simulink model "AplysiaFeedingSimulation - Copy"  (R2019b)
settings: Solver=FixedStepAuto  StartTime=0.0  StopTime=40  FixedStep=0.05  RelTol=1e-3
values from neighbouring files (symbols this model uses):
  A_hinge_Init = 0.05    [AplysiaFeedingNew.m]
  A_I2_Init = 0.05    [AplysiaFeedingNew.m]
  A_I3_anterior_Init = 0.05    [AplysiaFeedingNew.m]
  A_I3_Init = 0.05    [AplysiaFeedingNew.m]
  A_I4_Init = 0.05    [AplysiaFeedingNew.m]
  B20_Init = 0    [AplysiaFeedingNew.m]
  B31B32_Init = 1    [AplysiaFeedingNew.m]
  B38_Init = 1    [AplysiaFeedingNew.m]
  B40B30_Init = 0    [AplysiaFeedingNew.m]
  B4B5_Init = 0    [AplysiaFeedingNew.m]
  B64_Init = 0    [AplysiaFeedingNew.m]
  B6B9B3_Init = 0    [AplysiaFeedingNew.m]
  B7_Init = 0    [AplysiaFeedingNew.m]
  B8_Init = 0    [AplysiaFeedingNew.m]
  c_g = 1.0    (= 1)    [AplysiaFeedingNew.m]
  c_h = 1.0    (= 1)    [AplysiaFeedingNew.m]
  CBI2_Init = 1    [AplysiaFeedingNew.m]
  CBI3_Init = 0    [AplysiaFeedingNew.m]
  CBI4_Init = 0    [AplysiaFeedingNew.m]
  fixation_type_final = 10000    [AplysiaFeedingNew.m]
  fixation_type_initial = 10000    [AplysiaFeedingNew.m]
  K_sp_g = 0.1    [AplysiaFeedingNew.m]
  K_sp_h = 2.0    (= 2)    [AplysiaFeedingNew.m]
  max_hinge = 0.2    [AplysiaFeedingNew.m]
  max_I2 = 1.5    [AplysiaFeedingNew.m]
  max_I3 = 1    [AplysiaFeedingNew.m]
  max_I3ant = 0.6    [AplysiaFeedingNew.m]
  max_I4 = 1.75    [AplysiaFeedingNew.m]
  MCC_Init = 1    [AplysiaFeedingNew.m]
  mu_k_g = 0.3    [AplysiaFeedingNew.m]
  mu_k_h = 0.3    [AplysiaFeedingNew.m]
  mu_s_g = 0.4    [AplysiaFeedingNew.m]
  mu_s_h = 0.3    [AplysiaFeedingNew.m]
  P_I3_anterior_Init = 0    [AplysiaFeedingNew.m]
  P_I4_Init = 0    [AplysiaFeedingNew.m]
  postActivityExcitation_B40B30 = 3    [AplysiaFeedingNew.m]
  seaweed_strength = 10    [AplysiaFeedingNew.m]
  sens_chemical_lips_final = 10000    [AplysiaFeedingNew.m]
  sens_chemical_lips_initial = 10000    [AplysiaFeedingNew.m]
  sens_mechanical_grasper_final = 10000    [AplysiaFeedingNew.m]
  sens_mechanical_grasper_initial = 10000    [AplysiaFeedingNew.m]
  sens_mechanical_lips_final = 10000    [AplysiaFeedingNew.m]
  sens_mechanical_lips_initial = 10000    [AplysiaFeedingNew.m]
  sensory_trigger_time = 10000    [AplysiaFeedingNew.m]
  stim_B4B5_trigger_time_end = 10000    [AplysiaFeedingNew.m]
  stim_B4B5_trigger_time_start = 10000    [AplysiaFeedingNew.m]
  stim_CBI2_trigger_time_end = 10000    [AplysiaFeedingNew.m]
  stim_CBI2_trigger_time_start = 10000    [AplysiaFeedingNew.m]
  T_hinge_Init = 0    [AplysiaFeedingNew.m]
  T_I2_Init = 0.05    [AplysiaFeedingNew.m]
  T_I3_Init = 0.05    [AplysiaFeedingNew.m]
  tau_hinge = 1.0/sqrt(2)    [AplysiaFeedingNew.m]
  tau_I2_egestion = 1.4*1/sqrt(2)    [AplysiaFeedingNew.m]
  tau_I2_ingestion = 0.5*1/sqrt(2)    [AplysiaFeedingNew.m]
  tau_I3 = 1.0/sqrt(2)    [AplysiaFeedingNew.m]
  tau_I3anterior = 2.0/sqrt(2)    [AplysiaFeedingNew.m]
  tau_I4 = 1.0/sqrt(2)    [AplysiaFeedingNew.m]
  thresh_B31_bite_off = 0.55    [AplysiaFeedingNew.m]
  thresh_B31_bite_on = 0.9    [AplysiaFeedingNew.m]
  thresh_B31_reject_off = 0.6    [AplysiaFeedingNew.m]
  thresh_B31_reject_on = 0.89    [AplysiaFeedingNew.m]
  thresh_B31_swallow_off = 0.4    [AplysiaFeedingNew.m]
  thresh_B31_swallow_on = 0.75    [AplysiaFeedingNew.m]
  thresh_B4B5_protract = 0.7    [AplysiaFeedingNew.m]
  thresh_B64_bite_protract = 0.89    [AplysiaFeedingNew.m]
  thresh_B64_reject_protract = 0.5    [AplysiaFeedingNew.m]
  thresh_B64_swallow_protract = 0.4    [AplysiaFeedingNew.m]
  thresh_B6B9B3_bite_pressure = 0.2    [AplysiaFeedingNew.m]
  thresh_B6B9B3_reject_pressure = 0.75    [AplysiaFeedingNew.m]
  thresh_B6B9B3_swallow_pressure = 0.25    [AplysiaFeedingNew.m]
  unbroken_Init = 1    [AplysiaFeedingNew.m]
  use_hypothesized_connections = 0    [AplysiaFeedingNew.m]
  x_g_Init = 0.1    [AplysiaFeedingNew.m]
  x_gh_ref = 0.4    [AplysiaFeedingNew.m]
  x_h_Init = 0    [AplysiaFeedingNew.m]
  x_h_ref = 0.0    (= 0)    [AplysiaFeedingNew.m]
(part 2 of 2)

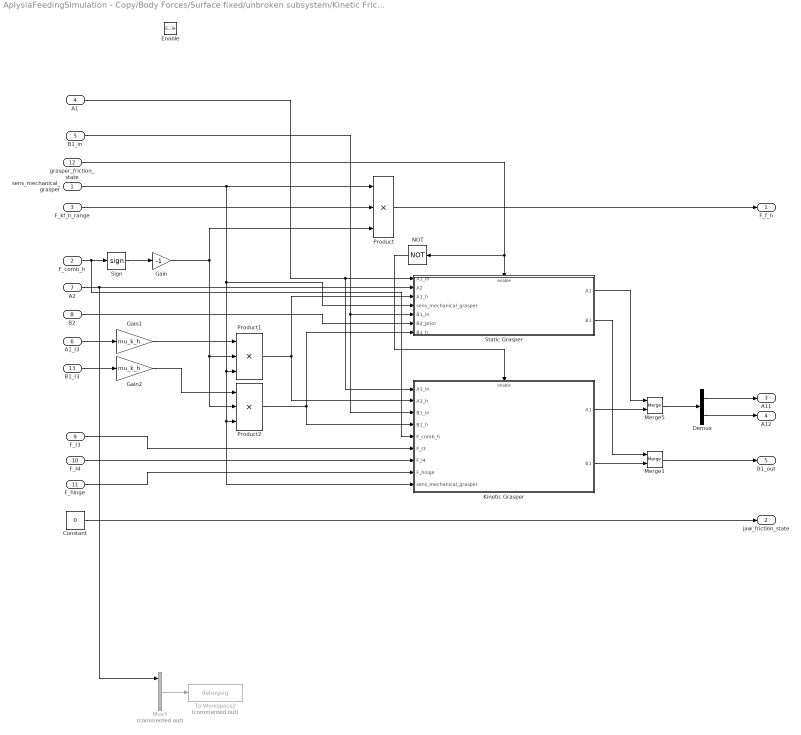
== system AplysiaFeedingSimulation - Copy/Body Forces/Surface fixed/unbroken subsystem/Kinetic Friction Behavior ==
  sens_mechanical_grasper : Inport
  F_comb_h : Inport  Port=2
  F_kf_h_range : Inport  Port=3
  A1 : Inport  Port=4
  B1_in : Inport  Port=5
  A1_I3 : Inport  Port=6
  A2 : Inport  Port=7
  B2 : Inport  Port=8
  F_I3 : Inport  Port=9
  F_I4 : Inport  Port=10
  F_hinge : Inport  Port=11
  grasper_friction_state : Inport  Port=12
  B1_I3 : Inport  Port=13
  Enable : EnablePort
  Constant : Constant  Value=0
  Demux : Demux  Outputs=2
  Gain : Gain  Gain=-1
  Gain1 : Gain  Gain=mu_k_h
  Gain2 : Gain  Gain=mu_k_h
  Kinetic Grasper : Subsystem
  Merge1 : Merge
  Merge5 : Merge
  Mux3 : Mux  Commented=on
  NOT : Logic  Operator=NOT  IconShape=distinctive  AllPortsSameDT=off  OutDataTypeStr=boolean
  Product : Product  Inputs=3
  Product1 : Product  Inputs=3
  Product2 : Product  Inputs=3
  Sign : Signum
  Static Grasper : Subsystem
  To Workspace2 : ToWorkspace  Commented=on  VariableName=debugsig  SaveFormat=Structure With Time  SampleTime=-1
  F_f_h : Outport
  jaw_friction_state : Outport  Port=2
  A11 : Outport  Port=3
  A12 : Outport  Port=4
  B1_out : Outport  Port=5
  wires:
  Constant/1 -> jaw_friction_state/1
  F_comb_h/1 -> Kinetic Grasper/5(F_comb_h), Sign/1
  Product/1 -> F_f_h/1
  F_kf_h_range/1 -> Product/2
  sens_mechanical_grasper/1 -> Static Grasper/4(sens_mechanical_grasper), Kinetic Grasper/9(sens_mechanical_grasper), Product2/3, Product1/3, Product/1
  Sign/1 -> Gain/1
  Gain/1 -> Product2/2, Product1/2, Product/3
  A1_I3/1 -> Gain1/1
  Gain1/1 -> Product1/1
  Merge5/1 -> Demux/1
  Demux/1 -> A11/1
  Demux/2 -> A12/1
  Static Grasper/1(A1) -> Merge5/1
  Kinetic Grasper/1(A1) -> Merge5/2
  Merge1/1 -> B1_out/1
  Kinetic Grasper/2(B1) -> Merge1/2
  Static Grasper/2(B1) -> Merge1/1
  A1/1 -> Kinetic Grasper/1(A1_in), Static Grasper/1(A1_in)
  B1_in/1 -> Static Grasper/5(B1_in), Kinetic Grasper/3(B1_in)
  B2/1 -> Static Grasper/6(B2_prior)
  F_hinge/1 -> Kinetic Grasper/8(F_hinge)
  F_I4/1 -> Kinetic Grasper/7(F_I4)
  F_I3/1 -> Kinetic Grasper/6(F_I3)
  grasper_friction_state/1 -> NOT/1, Static Grasper/Enable
  NOT/1 -> Kinetic Grasper/Enable
  Product1/1 -> Kinetic Grasper/2(A1_h), Static Grasper/3(A1_h)
  B1_I3/1 -> Gain2/1
  Gain2/1 -> Product2/1
  Product2/1 -> Kinetic Grasper/4(B1_h), Static Grasper/7(B1_h)
  Mux3/1 -> To Workspace2/1
  A2/1 -> Mux3/1, Static Grasper/2(A2)

== system AplysiaFeedingSimulation - Copy/Body Forces/Surface fixed/unbroken subsystem/Static Friction Behavior ==
  sens_mechanical_grasper : Inport
  F_comb_h : Inport  Port=2
  Enable : EnablePort
  Constant : Constant
  Constant1 : Constant  Value=0
  Gain : Gain  Gain=-1
  Product1 : Product
  F_f_h : Outport
  jaw_friction_state : Outport  Port=2
  A11 : Outport  Port=3
  A12 : Outport  Port=4
  B1 : Outport  Port=5
  wires:
  Constant/1 -> jaw_friction_state/1
  Constant1/1 -> A11/1, A12/1, B1/1
  Product1/1 -> F_f_h/1
  F_comb_h/1 -> Product1/2
  Gain/1 -> Product1/1
  sens_mechanical_grasper/1 -> Gain/1

== system AplysiaFeedingSimulation - Copy/Grasper Forces/Surface fixed/broken subsystem/Kinetic Friction Behavior ==
  sens_mechanical_grasper : Inport
  F_comb : Inport  Port=2
  F_kf_range : Inport  Port=3
  Enable : EnablePort
  Abs : Abs
  Constant : Constant  Value=0
  Divide : Product  Inputs=*/
  Gain : Gain  Gain=-1
  Product : Product
  Product1 : Product
  F_f_g : Outport
  grasper_friction_state : Outport  Port=2
  wires:
  Constant/1 -> grasper_friction_state/1
  F_kf_range/1 -> Product/2
  F_comb/1 -> Abs/1, Gain/1
  Gain/1 -> Divide/1
  Abs/1 -> Divide/2
  Divide/1 -> Product1/2
  Product/1 -> Product1/1
  Product1/1 -> F_f_g/1
  sens_mechanical_grasper/1 -> Product/1

== system AplysiaFeedingSimulation - Copy/Grasper Forces/Surface fixed/broken subsystem/Static Friction Behavior ==
  sens_mechanical_grasper : Inport
  F_comb : Inport  Port=2
  Enable : EnablePort
  Constant : Constant
  Gain : Gain  Gain=-1
  Product : Product
  F_f_g : Outport
  grasper_friction_state : Outport  Port=2
  wires:
  Constant/1 -> grasper_friction_state/1
  sens_mechanical_grasper/1 -> Gain/1
  F_comb/1 -> Product/2
  Gain/1 -> Product/1
  Product/1 -> F_f_g/1

== system AplysiaFeedingSimulation - Copy/Grasper Forces/Surface fixed/unbroken subsystem/Kinetic Friction Behavior ==
  sens_mechanical_grasper : Inport
  F_comb : Inport  Port=2
  F_kf_range : Inport  Port=3
  A2 : Inport  Port=4
  B2_in : Inport  Port=5
  Enable : EnablePort
  Add : Sum
  Constant : Constant  Value=0
  Demux : Demux  Outputs=2
  Gain : Gain  Gain=-1
  Gain1 : Gain  Gain=1 / c_g
  Product : Product
  Product1 : Product
  Reshape : Reshape  OutputDimensionality=Customize
  Sign : Signum
  F_f_g : Outport
  grasper_friction_state : Outport  Port=2
  A21 : Outport  Port=3
  A22 : Outport  Port=4
  B2_out : Outport  Port=5
  wires:
  Constant/1 -> grasper_friction_state/1
  F_kf_range/1 -> Product/2
  F_comb/1 -> Sign/1
  sens_mechanical_grasper/1 -> Product/1
  Demux/1 -> A21/1
  A2/1 -> Demux/1
  Demux/2 -> A22/1
  Sign/1 -> Gain/1
  B2_in/1 -> Add/1
  Gain1/1 -> Add/2
  Add/1 -> B2_out/1
  Gain/1 -> Product1/2
  Product/1 -> Product1/1
  Reshape/1 -> Gain1/1, F_f_g/1
  Product1/1 -> Reshape/1

== system AplysiaFeedingSimulation - Copy/Grasper Forces/Surface fixed/unbroken subsystem/Static Friction Behavior ==
  sens_mechanical_grasper : Inport
  F_comb : Inport  Port=2
  Enable : EnablePort
  Constant : Constant
  Constant1 : Constant  Value=0
  Gain : Gain  Gain=-1
  Product1 : Product
  F_f_g : Outport
  grasper_friction_state : Outport  Port=2
  A21 : Outport  Port=3
  A22 : Outport  Port=4
  B2 : Outport  Port=5
  wires:
  Constant/1 -> grasper_friction_state/1
  Constant1/1 -> A21/1, A22/1, B2/1
  Product1/1 -> F_f_g/1
  F_comb/1 -> Product1/2
  Gain/1 -> Product1/1
  sens_mechanical_grasper/1 -> Gain/1

== system AplysiaFeedingSimulation - Copy/Body Forces/Surface fixed/unbroken subsystem/Kinetic Friction Behavior/Kinetic Grasper ==
  A1_in : Inport
  A1_h : Inport  Port=2
  B1_in : Inport  Port=3
  B1_h : Inport  Port=4
  F_comb_h : Inport  Port=5
  F_I3 : Inport  Port=6
  F_I4 : Inport  Port=7
  F_hinge : Inport  Port=8
  sens_mechanical_grasper : Inport  Port=9
  Enable : EnablePort
  Add : Sum  Inputs=+--  InputSameDT=on
  Add1 : Sum
  Add2 : Sum
  Add3 : Sum
  Gain : Gain  Gain=-1
  Gain1 : Gain  Gain=1 / c_h
  Gain2 : Gain  Gain=1 / c_h
  Gain3 : Gain  Gain=mu_k_g
  Product : Product  Inputs=3
  Sign : Signum
  A1 : Outport
  B1 : Outport  Port=2
  wires:
  A1_h/1 -> Gain2/1
  Gain2/1 -> Add1/2
  A1_in/1 -> Add1/1
  Add1/1 -> A1/1
  F_comb_h/1 -> Add/1
  Add/1 -> Sign/1
  Sign/1 -> Gain/1
  Gain/1 -> Product/2
  Gain3/1 -> Product/3
  sens_mechanical_grasper/1 -> Product/1
  B1_h/1 -> Add2/1
  Add2/1 -> Gain1/1
  Gain1/1 -> Add3/2
  B1_in/1 -> Add3/1
  Add3/1 -> B1/1
  F_I3/1 -> Add/2
  F_hinge/1 -> Add/3
  Product/1 -> Add2/2
  F_I4/1 -> Gain3/1

== system AplysiaFeedingSimulation - Copy/Body Forces/Surface fixed/unbroken subsystem/Kinetic Friction Behavior/Static Grasper ==
  A1_in : Inport
  A2 : Inport  Port=2
  A1_h : Inport  Port=3
  sens_mechanical_grasper : Inport  Port=4
  B1_in : Inport  Port=5
  B2_prior : Inport  Port=6
  B1_h : Inport  Port=7
  Enable : EnablePort
  Add{,1..3} (4 alike) : Sum
  Gain : Gain  Gain=c_g
  Gain1 : Gain  Gain=-1
  Gain2 : Gain  Gain=1 / c_h
  Gain3 : Gain  Gain=c_g
  Gain4 : Gain  Gain=1 / c_h
  Product : Product
  Product1 : Product
  A1 : Outport
  B1 : Outport  Port=2
  wires:
  A2/1 -> Gain/1
  sens_mechanical_grasper/1 -> Gain1/1
  Gain1/1 -> Product1/1, Product/1
  Gain/1 -> Product/2
  Product/1 -> Add/1
  A1_h/1 -> Add/2
  Add/1 -> Gain2/1
  Gain2/1 -> Add1/2
  A1_in/1 -> Add1/1
  Add1/1 -> A1/1
  B2_prior/1 -> Gain3/1
  Gain3/1 -> Product1/2
  Product1/1 -> Add2/1
  B1_h/1 -> Add2/2
  Add2/1 -> Gain4/1
  Gain4/1 -> Add3/2
  B1_in/1 -> Add3/1
  Add3/1 -> B1/1

== matlab function AplysiaFeedingSimulation - Copy/neural_comp ==
  data: use_hypothesized_connections input; thresh_B64 input; thresh_B4B5_protract input; thresh_B31 input; thresh_B6B9B3 input; tau input; MCC_In input; y output; sens_mechanical_lips input; sens_chemical_lips input; sens_mechanical_grasper input; stim_B4B5 input; stim_CBI2 input; CBI2_In input; CBI3_In input; CBI4_In input; B64_In input; B4B5_In input; B20_In input; B40B30_In input; B31B32_In input; B6B9B3_In input; B8_In input; P_I4_In input; A_I4_in input; P_I3_anterior_In input; A_I3_anterior_In input; T_I3_In input; A_I3_In input; T_I2_In input; A_I2_In input; T_hinge_In input; A_hinge_In input; x_gh input; B7_In input; B38_In input
% function y = fcn(x_gh, MCC_In, CBI2_In, T_I3_In,... 
% use_hypothesized_connections, stim_CBI2, B64_In, sens_mechanical_lips,... 
% sens_chemical_lips, sens_mechanical_grasper, B4B5_In, CBI3_In,...
% thresh_B64_swallow_protract, thresh_B64_bite_protract, thresh_B64_reject_protract,...
% B31B32_In, stim_B4B5, thresh_B4B5_In_protract, CBI4_In, B40B30_In, P_I4_In,...
% thresh_B31_swallow_on, thresh_B31_swallow_off, thresh_B31_reject_on,...
% thresh_B31_reject_off,thresh_B31_bite_on,thresh_B31_bite_off,...
% thresh_B6B9B3_bite_pressure, thresh_B6B9B3_swallow_pressure,thresh_B6B9B3_reject_pressure,...
% B20_In, thresh_B7_reject_protract,thresh_B7_bite_protract,thresh_B38_retract,tau_I4,...
% A_I4_In,B8_In,P_I3_anterior_In,tau_I3anterior,A_I3_anterior_In,B38_In,B6B9B3_In,...
% tau_I3,A_I3_In,tau_I2_ingestion,tau_I2_egestion,A_I2_In,T_I2_In,tau_hinge,...
% A_hinge_In,T_hinge_In,B7_In,refractory_CBI3,postActivityExcitation_B40B30)

function y = fcn(use_hypothesized_connections, thresh_B64, thresh_B4B5_protract,...
    thresh_B31, thresh_B6B9B3, tau, MCC_In, sens_mechanical_lips, sens_chemical_lips,...
    sens_mechanical_grasper,stim_B4B5, stim_CBI2, CBI2_In, CBI3_In, CBI4_In,...
    B64_In, B4B5_In, B20_In, B40B30_In, B31B32_In,B6B9B3_In, B8_In, P_I4_In,...
    A_I4_in,P_I3_anterior_In, A_I3_anterior_In,T_I3_In, A_I3_In, T_I2_In, A_I2_In,...
    T_hinge_In, A_hinge_In, x_gh,...
    B7_In, B38_In)

%  %% Update Metacerebral cell: 
                % assume here feeding arousal continues
                % indefinitely, once started. 
                %{
                MCC is active IF
                    General Food arousal is on
                %}

                MCC_Out = MCC_In;
                
                B64_Out = B64_In;
                B4B5_Out = B4B5_In;
%                 B31B32_Out = B31B32_In; % WRONG
                B7_Out = B7_In; % WRONG
                B38_Out = B38_In; % WRONG
                
                %% Update CBI-2
                %{
                CBI2 is active IF
                    MCC is on 
                    AND (
                        (Mechanical Stimulation at Lips AND Chemical Stimulation at Lips AND No mechanical stimuli in grasper)
                        OR 
                        (Mechanical in grasper and no Chemical Stimulation at Lips)
                        OR
                        (B4/B5 is firing strongly (>=2)))
                %}

                %CBI2 - updated 6/7/2020
                %with hypothesized connections from B4/B5
                if (use_hypothesized_connections ==1)
                     CBI2_Out = (stim_CBI2==0)*... if electrode above CBI-2 is off, do this:
                         MCC_In*(~B64_In)*((sens_mechanical_lips && sens_chemical_lips &&(~sens_mechanical_grasper))||(sens_mechanical_grasper &&(~sens_chemical_lips))||(B4B5_In>=2))+...
                         (stim_CBI2==1);
                else
                %without hypothesized connections from B4/B5
                    CBI2_Out = (stim_CBI2==0)*... if electrode above CBI-2 is off, do this:
                        MCC_In*(~B64_In)*((sens_mechanical_lips && sens_chemical_lips &&(~sens_mechanical_grasper))||(sens_mechanical_grasper&&(~sens_chemical_lips)))+...
                        (stim_CBI2==1);
                end

                %% Update CBI-3
                % requires stimuli_mech_last AND stimuli_chem_last
                %{
                CBI3 is active IF
                    MCC is on
                    AND
                    Mechanical Simulation at Lips
                    AND
                    Chemical Stimulation at Lips
                    AND
                    B4/B5 is NOT firing strongly
                    AND
                    CBI3 is NOT in a refractory period
                %}

                %CBI3 can experieince a refractory period following strong inhibition from B4/B5
                %check if a refractory period is occuring

%             %modified to only turn on refreactory after the strong stimulation
%                 if((B4B5_In>=2) && (CBI3_stimON==0))
%                    CBI3_stimON = j;   
%                    %CBI3_refractory = 1;
%                 end
%                 if ((CBI3_stimON ~=0) && (B4B5_In<2))
%                    CBI3_refractory = 1;
%                    CBI3_stimOFF = j;  
%                    CBI3_stimON = 0;    
%                 end 
% 
%                 if(CBI3_refractory && j<(CBI3_stimOFF+refractory_CBI3/1000/obj.TimeStep))
%                    CBI3_refractory = 1; 
%                 else
%                     CBI3_stimOFF = 0;
%                     CBI3_refractory = 0; 
%                 end
% 
% 
%                 %CBI3 - updated 6/7/2020    
%                 %with hypothesized connections from B4/B5    
%                 if (use_hypothesized_connections ==1)
%                     CBI3_Out = MCC_In*(sens_mechanical_lips*sens_chemical_lips)*((B4B5_In<2))*(~CBI3_refractory);   
%                 else
%                 %without hypothesized connections from B4/B5  
%                     CBI3_Out = MCC_In*(sens_mechanical_lips*sens_chemical_lips); 
%                 end

                CBI3_Out = MCC_In*(sens_mechanical_lips*sens_chemical_lips); 


                %% Update CBI4 - added 2/27/2020
                %{
                CBI4 is active IF  mediates swallowing and rejection
                    MCC is on
                    AND
                        (Mechanical Stimulation at Lips
                        OR
                        Chemical Stimulation at Lips)
                    AND
                    Mechanical Stimulation in grasper
                %}
                CBI4_Out = MCC_In*(sens_mechanical_lips || sens_chemical_lips)*sens_mechanical_grasper;

%                 %% Update B64
%                 % list of inputs
%                 % Protraction threshold excites
%                 % grasper pressure excites - still figuring out how to implement
%                 % retraction threshold inhibits
%                 % B31/32 inhibits
% 
%                 %If there is mechanical and chemical stimuli at the lips and there is
%                 %seaweed in the grasper -> swallow
% 
%                 %If there is mechanical and chemical stimuli at the lips and there is
%                 %NOT seaweed in the grasper -> bite
% 
%                 %If there is not chemical stimuli at the lips but there is mechanical
%                 %stimuli ->reject
% 
%                 %{
%                 B64 is active IF
%                     MCC is on
%                     AND
%                     IF CBI3 is active (ingestion)
%                         IF mechanical stimulation is in grasper (swallowing)
%                             Relative Grasper Position is Greater than B64 Swallowing Protraction threshold
%                         IF mechanical stimulation is NOT in grasper (biting)
%                             Relative Grasper Position is Greater than B64 Biting Protraction threshold
%                     IF CBI3 is NOT active (rejection)
%                         Relative Grasper Position is Greater than B64 Rejection Protraction threshold
%                     AND
%                     B31/B32 is NOT active
%                     AND
%                     IF CBI3 is active (ingestion)
%                         IF mechanical stimulation is in grasper (swallowing)
%                             NOT (Relative Grasper Position is less than B64 Swallow Retraction threshold)
%                         IF mechanical stimulation is NOT in grasper (biting)
%                             NOT(Relative Grasper Position is less than B64 Biting Retraction threshold)
%                     IF CBI3 is NOT active (rejection)
%                         NOT(Relative Grasper Position is less than B64 Rejection Retraction threshold)
%                 %}
% 
%                 B64_proprioception = (CBI3_In*(... % checks protraction threshold - original 0.5
%                                                 (  sens_mechanical_grasper *(x_gh>thresh_B64(2)))||...
%                                                 ((~sens_mechanical_grasper)*(x_gh>thresh_B64(1)))))...
%                                             ||...
%                                                 ((~CBI3_In)*(x_gh>thresh_B64(3)));
% 
%                 %B64
%                 B64_Out=MCC_In*(~B31B32_In)*B64_proprioception;

                %% Update B4/B5: 
                %{
                B4/B5 is active IF
                    MCC is ON
                    AND
                    IF stimulating electrode is off
                        Strongly firing IF CBI3 is NOT active (rejection)
                            AND
                            B64 is active (retraction)
                            AND
                            Relative grasper position is greater than B4/B5 threshold (early retraction)
                        weakly firing IF CBI3 is active (ingestion)
                            AND
                            B64 is active (retraction)
                            AND
                            mechanical stimulation is in grasper (swallowing)
                    If stimulating electrode is on
                        Activity is set to 2 to designate strong firing
                %}

                %B4B5_Out
%                 B4B5_Out=MCC_In*...
%                             ((~stim_B4B5)*... % when B4/B5 electrode is off
%                                 (2*(~CBI3_In)*...% if egestion
%                                     B64_In*(x_gh>thresh_B4B5_protract)) +... 
%                                 ((CBI3_In)*(sens_mechanical_grasper)*B64_In))... % if swallowing
%                     +2*stim_B4B5; % when B4/B5 electrode is on (and +1) then turn B4/B5 on to "emergency" mode

                %% Update B20 - updated 2/27/2020
                % Not active if CB1-3 is on (strongly inhibited)
                %excited by CBI2 but excitation is weaker than inhibition from CBI3
                %{
                (CBI2 is active
                    OR	
                    CBI4 is active
                    OR
                    B63 (B31/32) is active)
                        AND
                        CBI3 is NOT active
                        AND
                        B64 is NOT active

                %}
                B20_Out = MCC_In*((CBI2_In || CBI4_In) || B31B32_In)*(~CBI3_In)*(~B64_In);

               %% Update B40/B30
                %{
                B40/B30 is active IF
                    MCC is ON
                    AND
                    (CBI2 is active
                    OR 
                    CBI4 is active
                    OR 
                    B63 (B31/32) is active)
                    AND 
                    B64 is not active
                %}

                % B30/B40 have a fast inhibitory and slow excitatory connection with
                % B8a/b. To accomodate this, we track when B30/B40 goes from a active
                % state to a quiescent state 

                B40B30_Out = MCC_In*((CBI2_In || CBI4_In) || B31B32_In)*(~B64_In);

%                 %check if B30/B40 has gone from active to quiescent
%                 if((B40B30_In ==1) && (B40B30_Out==0))
%                    B40B30_offTime = j;
%                 end

                %% Update B31/B32: -updated 2/27/2020
                % activated if grasper retracted enough, inhibited if
                % pressure exceeds a threshold or grasper is protracted far enough
                %{
                B31/B32 is active IF
                    MCC is ON
                    AND
                    IF CBI3 is active (ingestion)
                        B64 is NOT active (protraction)
                        AND
                            Graper pressure is less than half of its maximum (open)
                            OR
                            CBI2 is active (biting)
                        AND
                        IF B31/B32 is NOT firing (switching to protraction)
                            The relative grasper position is less than the retraction threshold
                        IF B31/B32 is firing (protraction)
                            The relative grasper position is less than the protraction threshold
                    IF CBI3 is NOT active (rejection)
                        B64 is NOT active (protraction)
                        AND
                        Grasper Pressure is greater than a quarter of the maximum (closing or closed)
                        AND
                            CBI2 is active
                            OR
                            CBI4 is active
                        AND
                        IF B31/B32 is NOT firing (switching to protraction)
                            The relative grasper position is less than the retraction threshold
                        IF B31/B32 is firing (protraction)
                            The relative grasper position is less than the protraction threshold
                %}

                %B31/B32s thresholds may vary for different behaviors. These are set
                %here
                if (sens_mechanical_grasper && CBI3_In) %swallowing
                    on_thresh = thresh_B31(3);
                    off_thresh = thresh_B31(4);
                elseif (sens_mechanical_grasper && (~CBI3_In)) %rejection
                    on_thresh = thresh_B31(5);
                    off_thresh = thresh_B31(6);
                else %biting
                    on_thresh = thresh_B31(1);
                    off_thresh = thresh_B31(2);        
                end

                B31B32_Out=MCC_In*(...
                    CBI3_In*... %if ingestion
                        ((~B64_In)*((P_I4_In<(1/2))||CBI2_In)*... 
                            ((~B31B32_In)*(x_gh<off_thresh)+...
                               B31B32_In *(x_gh<on_thresh)))+...
                  (~CBI3_In)*... %if egestion
                        ((~B64_In)*(P_I4_In>(1/4))*(CBI2_In||CBI4_In)*...
                            ((~B31B32_In)*(x_gh<off_thresh)+...
                               B31B32_In *(x_gh<on_thresh))));

                %% Update B6/B9/B3: 
                % activate once pressure is high enough in ingestion, or low enough in
                % rejection
                %{
                NEW VERSION:
                B6/B9/B3 is active IF
                    MCC is active
                    AND
                    B4/B5 is NOT firing strongly
                    AND
                    IF CBI3 is active (ingestion)
                        B64 is active (retraction)
                        AND
                        Grasper pressure is greater than B6/B3/B9 pressure threshold (closed)
                    IF CBI3 is not active (rejection)
                        B64 is active (retraction)
                        AND
                        Grasper pressure is less than B6/B3/B9 pressure threshold (open)
                %}
                %{
                B6/B9/B3 is active IF
                    MCC is active
                    AND
                    B64 is active (retraction)
                    AND
                    B4/B5 is NOT firing strongly
                    AND (
                    (CBI3 is active (ingestion)
                     AND
                     There is NOT mechanical stimulation in mouth (biting)
                     AND
                     Grasper pressure is greater than B6/B3/B9 biting pressure
                     threshold (closed))
                    OR
                    (CBI3 is active (ingestion)
                     AND
                     There is mechanical stimulation in mouth (swallowing)
                     AND
                     Grasper pressure is greater than B6/B3/B9 swallowing pressure
                     threshold (closed))
                    OR
                    (CBI3 is NOT active (rejection)
                     AND
                     Grasper pressure is NOT greater than B6/B3/B9 rejection pressure
                     threshold (open))
                    )
                %}

                %B6/B9/B3
               B6B9B3_Out= MCC_In*B64_In*(~(B4B5_In>=2))*(...
                                (CBI3_In && ~sens_mechanical_grasper)*... biting
                                    (P_I4_In>thresh_B6B9B3(1))...
                                +...
                                (CBI3_In && sens_mechanical_grasper)*... swallowing
                                    (P_I4_In>thresh_B6B9B3(2))...
                                +...
                                (~CBI3_In)*... rejection
                                    (~(P_I4_In>thresh_B6B9B3(3))));

                %% Update B8a/b
                % active if excitation from B6/B9/B3 plus protracted
                % sensory feedback exceeds threshold of 1.9, and not inhibited by
                % either B31/B32 or by sensory feedback from being retracted. If B4/B5 is
                % highly excited (activation level is 2 instead of just 1) then shut
                % down B8a/b.
                %{
                B8a/b is active IF
                    MCC is on
                    AND
                        B64 is active
                        OR
                        B40/B30 is NOT active
                        OR
                        B20 is active
                    AND
                    B4/B5 is not active
                    AND
                        B20 is active
                        OR
                        B31/B32 is NOT active
                %}

                %B8a/b recieves slow exitatory input from B30/B40 functionally this
                %causes strong firing immediatly following B30/B40 cessation in biting
                %and swallowing
%                 if(B40B30_In==0 && j<(B40B30_offTime+postActivityExcitation_B40B30/1000/obj.TimeStep))
%                     B40B30_excite = 1; 
%                 else
%                     B40B30_excite = 0; 
%                 end
 
                %B8a/b - updated 5/25/2020   
                B8_Out = MCC_In*(~(B4B5_In>=2))*(...%B4/5 inhibits when strongly active
                            CBI3_In*(... % if ingestion
                                B20_In || (B40B30_In)*(~B31B32_In))+... %B4030 is already delayed
                            (~CBI3_In)*(... % if rejection
                                B20_In));

%                 %% Update B7 - ONLY ACTIVE DURING EGESTION and BITING
%                 % turn on as you get to peak protraction
%                 %in biting this has a threshold that it stops applying effective force -
%                 %biomechanics
%                 %{
%                 B7 is active IF
%                     ((CBI3 is NOT active (rejection)
%                     OR
%                     There is mechanical stimulation in mouth
%                     AND
%                         (The relative position of the grasper is greater than the rejection protraction threshold
%                         OR
%                         Grasper pressure is very high) (closed))
%                     OR
%                     (CBI3 is active
%                     AND
%                     There is NOT mechanical stimulation in mouth (biting)
%                     AND
%                         (The relative position of the grasper is greater than the bite protraction threshold
%                         OR
%                         Grasper pressure is very high) (closed))
%                 %}
%                 B7_Out = MCC_In*( ...
%                                   (((~CBI3_In) ||  (sens_mechanical_grasper))*((x_gh>=thresh_B7_reject_protract)||(P_I4_In>(.97)))) + ...
%                                   (  (CBI3_In  && (~sens_mechanical_grasper))*((x_gh>=thresh_B7_bite_protract)  ||(P_I4_In>(.97)))) ...
%                                   );
% 
%                 %% Update B38: 
%                 % If already active, remain active until protracted past
%                 % 0.5.  If inactive, become active if retracted to 0.1 or further. 
%                 %{
%                 B38 is active IF
%                     MCC is ON
%                     AND
%                     mechanical stimulation in the grasper (swallowing or rejection)
%                     AND
%                     IF CBI3 is active (ingestion)
%                         Relative grasper position is less than B38 ingestion threshold
%                     IF CBI3 is not active (rejection)
%                         Turn off B38
%                 %}
% 
%                 %B38
% 
%                 B38_Out=MCC_In*(sens_mechanical_grasper)*(...
%                     (CBI3_In)*(... % if CBI3 active do the following:
%                         ((x_gh)<thresh_B38_retract)));
% 
                %% Update I4: If food present, and grasper closed, then approaches
                % pmax pressure as dp/dt=(B8*pmax-p)/tau_p.  Use a quasi-backward-Euler
                
                P_I4_Out = (A_I4_in - P_I4_In) / tau(1);
                A_I4_Out = (B8_In - A_I4_in) / tau(1);
                  
                %% Update pinch force: If food present, and grasper closed, then approaches
                % pmax pressure as dp/dt=(B8*pmax-p)/tau_p.  Use a quasi-backward-Euler

                Bcomp = B38_In + B6B9B3_In;
                P_I3_anterior_Out = (A_I3_anterior_In - P_I3_anterior_In) / tau(2);
                A_I3_anterior_Out = (Bcomp - A_I3_anterior_In) / tau(2);
                
                %% Update I3 (retractor) activation: dm/dt=(B6-m)/tau_m

                T_I3_Out = (A_I3_In - T_I3_In) / tau(3);
                A_I3_Out = (B6B9B3_In - A_I3_In) / tau(3);
                
                %% Update I2 (protractor) activation: dm/dt=(B31-m)/tau_m.  quasi-B-Eul.

                tau_I2 = tau(4)*CBI3_In + tau(5)*(1-CBI3_In);
                T_I2_Out = (A_I2_In - T_I2_In) / tau_I2;
                A_I2_Out = (B31B32_In - A_I2_In) / tau_I2;
                
                
                %% Update Hinge activation: dm/dt=(B7-m)/tau_m.  quasi-B-Eul.
                %bvec(12,j+1)=(tau_m*hinge_last+dt*B7_last)/(tau_m+dt);%old

                T_hinge_Out = (A_hinge_In - T_hinge_In) / tau(6);
                A_hinge_Out = (B7_In - A_hinge_In) / tau(6);

% y = [MCC_Out, CBI2_Out, T_I3_Out, CBI3_Out, CBI4_Out, B64_Out, B4B5_Out, B20_Out, B40B30_Out, B31B32_Out,...
%     B6B9B3_Out, B8_Out, B7_Out, B38_Out, P_I4_Out,A_I4_Out,P_I3_anterior_Out,A_I3_anterior_Out,A_I3_Out,...
%     T_I2_Out,A_I2_Out,T_hinge_Out,A_hinge_Out]; %23 outputs

y = [MCC_Out, CBI2_Out, CBI3_Out, CBI4_Out, B64_Out, B4B5_Out, B20_Out,...
    B40B30_Out, B31B32_Out, B6B9B3_Out, B8_Out, P_I4_Out, A_I4_Out,...
    P_I3_anterior_Out,A_I3_anterior_Out,T_I3_Out, A_I3_Out, T_I2_Out,... 
    A_I2_Out, T_hinge_Out,A_hinge_Out,...
    B7_Out, B38_Out]; %23 outputs
